simulink model "threePulse"  (Simulink 7.5)
settings: Solver=ode45  StartTime=0.0  StopTime=0.1  RelTol=1e-3
undefined symbols (not defined in the file): deg
libraries: powerlib x14, powerlib_extras x4
settings Model: Creator=Singhal  LastModifiedBy=Singhal

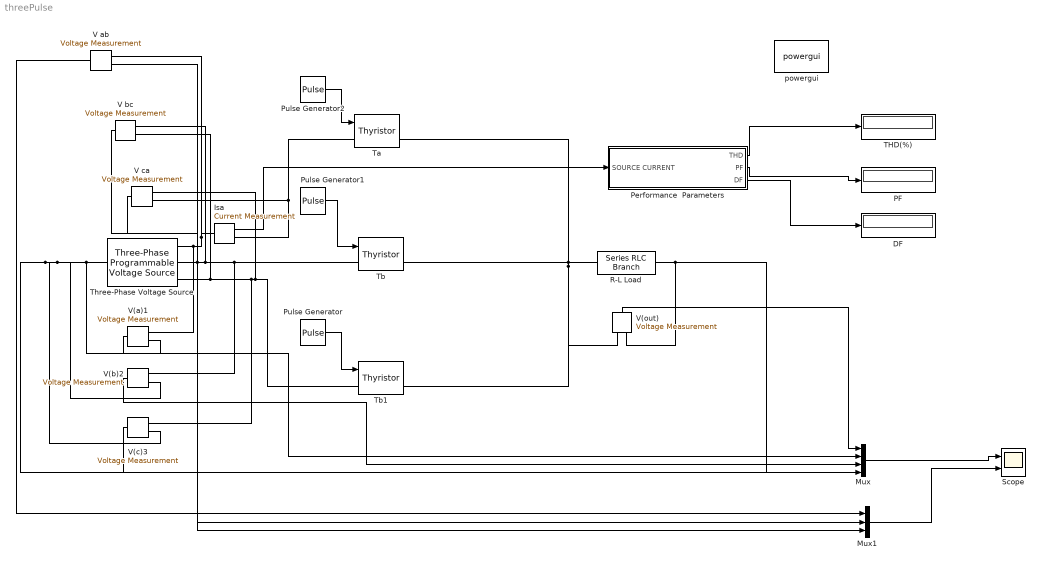
== system threePulse ==
  DF : Display
  Isa : powerlib/Measurements/Current Measurement  DialogController=POWERSYS.PowerSysDialog  SystemSampleTime=-1  PhasorSimulation=off  OutputType=Complex  PSBequivalent=0
  Mux : Mux
  Mux1 : Mux  Inputs=3
  PF : Display
  Performance  Parameters : Subsystem
  Pulse Generator : DiscretePulseGenerator  PulseType=Time based  Amplitude=1  Period=0.02  PulseWidth=5  PhaseDelay=(deg+270)/18000  SampleTime=1
  Pulse Generator1 : DiscretePulseGenerator  PulseType=Time based  Amplitude=1  Period=0.02  PulseWidth=5  PhaseDelay=(deg+150)/18000  SampleTime=1
  Pulse Generator2 : DiscretePulseGenerator  PulseType=Time based  Amplitude=1  Period=0.02  PulseWidth=5  PhaseDelay=(deg+30)/18000  SampleTime=1
  R-L Load : powerlib/Elements/Series RLC Branch  DialogController=POWERSYS.PowerSysDialog  PhysicalDomain=powersysdomain  SubClassName=unknown  LeftPortType=p1  RightPortType=p1  LConnTagsString=__new0  RConnTagsString=__new0  BranchType=RL  Resistance=1  Inductance=1e-3  SetiL0=off  InitialCurrent=0  Capacitance=1e-6  Setx0=off  InitialVoltage=0  Measurements=None
  Scope : Scope  NumInputPorts=2
      settings: YMin=-90~-150  YMax=90~150
  THD(%) : Display
  Ta : powerlib/Power Electronics/Thyristor  DialogController=POWERSYS.PowerSysDialog  SystemSampleTime=-1  Ron=0.001  Lon=0  Vf=0.8  IC=0  Rs=500  Cs=250e-9  Measurements=on
  Tb : powerlib/Power Electronics/Thyristor  DialogController=POWERSYS.PowerSysDialog  SystemSampleTime=-1  Ron=0.001  Lon=0  Vf=0.8  IC=0  Rs=500  Cs=250e-9  Measurements=on
  Tb1 : powerlib/Power Electronics/Thyristor  DialogController=POWERSYS.PowerSysDialog  SystemSampleTime=-1  Ron=0.001  Lon=0  Vf=0.8  IC=0  Rs=500  Cs=250e-9  Measurements=on
  Three-Phase Voltage Source : powerlib/Electrical Sources/Three-Phase Programmable Voltage Source  DialogController=POWERSYS.PowerSysDialog  SystemSampleTime=-1  PositiveSequence="[100  0 50]"  VariationEntity=None  VariationType=Step  VariationStep=0.5  VariationRate=10  VariationMagnitude=0.3  VariationFrequency=2  VariationTiming=[1 2]  VariationPhaseA=off  Amplitudes=[1 0.8 1.2 1.0]  TimeValues=[0 0.1 0.15 0.2]  HarmonicGeneration=off  HarmonicA=[3 0.2 -25 0]  HarmonicB=[2 0.15 35 2]  Timing="[0.05  3]"
  V ab : powerlib/Measurements/Voltage Measurement  DialogController=POWERSYS.PowerSysDialog  SystemSampleTime=-1  PhasorSimulation=off  OutputType=Complex  PSBequivalent=0
  V bc : powerlib/Measurements/Voltage Measurement  DialogController=POWERSYS.PowerSysDialog  SystemSampleTime=-1  PhasorSimulation=off  OutputType=Complex  PSBequivalent=0
  V ca : powerlib/Measurements/Voltage Measurement  DialogController=POWERSYS.PowerSysDialog  SystemSampleTime=-1  PhasorSimulation=off  OutputType=Complex  PSBequivalent=0
  V(a)1 : powerlib/Measurements/Voltage Measurement  DialogController=POWERSYS.PowerSysDialog  SystemSampleTime=-1  PhasorSimulation=off  OutputType=Complex  PSBequivalent=0
  V(b)2 : powerlib/Measurements/Voltage Measurement  DialogController=POWERSYS.PowerSysDialog  SystemSampleTime=-1  PhasorSimulation=off  OutputType=Complex  PSBequivalent=0
  V(c)3 : powerlib/Measurements/Voltage Measurement  DialogController=POWERSYS.PowerSysDialog  SystemSampleTime=-1  PhasorSimulation=off  OutputType=Complex  PSBequivalent=0
  V(out) : powerlib/Measurements/Voltage Measurement  DialogController=POWERSYS.PowerSysDialog  SystemSampleTime=-1  PhasorSimulation=off  OutputType=Complex  PSBequivalent=0
  powergui : powerlib/powergui  Priority=1  SystemSampleTime=-1  SimulationMode=Continuous  SampleTime=50e-6  frequency=60  SPID=off  DisableSnubberDevices=off  DisableRonSwitches=off  DisableVfSwitches=off  SwTol=0  Interpol=off  frequencyindice=50  echomessages=off  HookPort=off  DisplayEquations=off  FunctionMessages=off  EnableUseOfTLC=off  x0status=blocks  RestoreLinks=warning  ResistiveCurrentMeasurement=off  Ylog=off  Xlog=on  ShowGrid=off  save=off  variable=ZData  ZoomFFT=off  StartTime=0.0  cycles=1  DisplayStyle=1  FreqAxis=off  MaxFrequency=1000  frequencyindicesteady=1  display=off  methode=off
  wires:
  Pulse Generator/1 -> Tb1/1
  Pulse Generator1/1 -> Tb/1
  Pulse Generator2/1 -> Ta/1
  Performance  Parameters/2(PF) -> PF/1
  Performance  Parameters/3(DF) -> DF/1
  Performance  Parameters/1(THD) -> THD(%)/1
  Isa/1 -> Performance  Parameters/1(SOURCE CURRENT)
  V(out)/1 -> Mux/1
  V(a)1/1 -> Mux/2
  V(b)2/1 -> Mux/3
  V(c)3/1 -> Mux/4
  Mux/1 -> Scope/1
  V ab/1 -> Mux1/1
  V bc/1 -> Mux1/2
  V ca/1 -> Mux1/3
  Mux1/1 -> Scope/2
  connections:
  Three-Phase Voltage Source/LConn1 -- V(a)1/LConn2 -- V(b)2/LConn2 -- R-L Load/RConn1 -- V(out)/LConn2 -- V(c)3/LConn2
  Tb1/RConn1 -- R-L Load/LConn1 -- Ta/RConn1 -- Tb/RConn1 -- V(out)/LConn1
  Tb/LConn1 -- V(b)2/LConn1 -- Three-Phase Voltage Source/RConn2 -- V ab/LConn2 -- V bc/LConn1
  Tb1/LConn1 -- V(c)3/LConn1 -- Three-Phase Voltage Source/RConn3 -- V bc/LConn2 -- V ca/LConn1
  Isa/LConn1 -- Three-Phase Voltage Source/RConn1 -- V(a)1/LConn1 -- V ab/LConn1
  Isa/RConn1 -- Ta/LConn1 -- V ca/LConn2

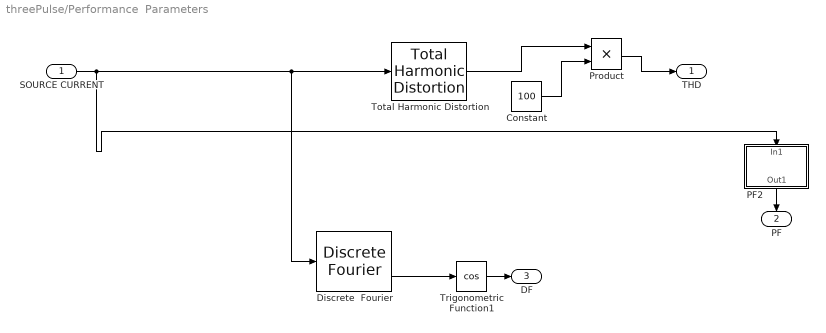
== system threePulse/Performance  Parameters ==
  SOURCE CURRENT : Inport
  Constant : Constant  Value=100  OutDataType=fixdt(1, 16)  OutScaling=2^0
  Discrete  Fourier : powerlib_extras/Discrete Measurements/Discrete  Fourier  DialogController=POWERSYS.PowerSysDialog  SystemSampleTime=-1  Freq=50  n=1  Par_Init=[0 0]  Ts=50e-6
  PF2 : Subsystem
  Product : Product  OutDataType=fixdt(1, 16)  OutScaling=2^0  RndMeth=Zero
  Total Harmonic Distortion : powerlib_extras/Measurements/Total Harmonic Distortion  DialogController=POWERSYS.PowerSysDialog  SystemSampleTime=-1  f1=50
  Trigonometric Function1 : Trigonometry  Operator=cos
  THD : Outport
  PF : Outport  Port=2
  DF : Outport  Port=3
  wires:
  SOURCE CURRENT/1 -> PF2/1(In1), Discrete  Fourier/1, Total Harmonic Distortion/1
  Discrete  Fourier/2 -> Trigonometric Function1/1
  PF2/1(Out1) -> PF/1
  Trigonometric Function1/1 -> DF/1
  Constant/1 -> Product/2
  Total Harmonic Distortion/1 -> Product/1
  Product/1 -> THD/1

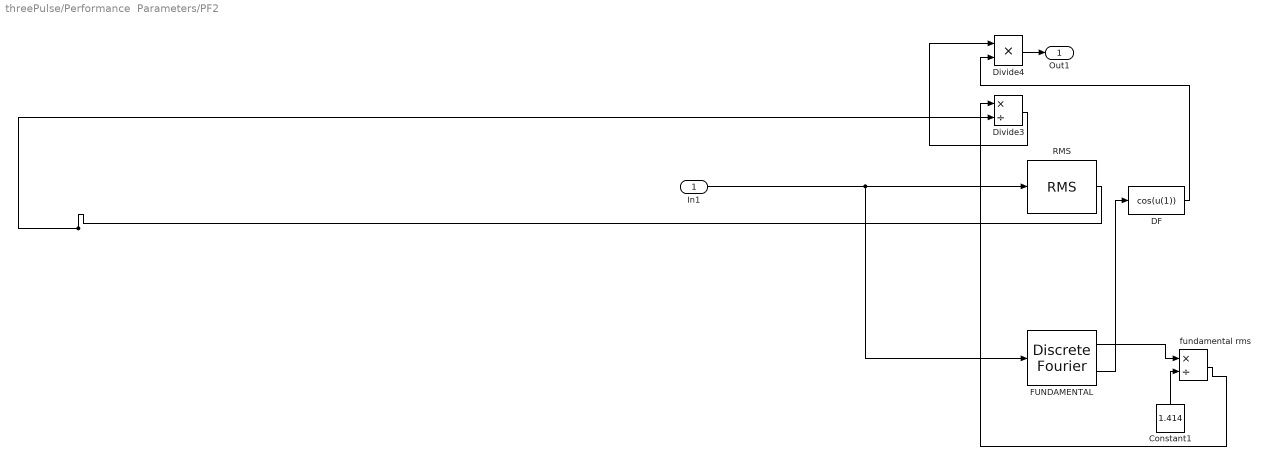
== system threePulse/Performance  Parameters/PF2 ==
  In1 : Inport
  Constant1 : Constant  Value=1.414  OutDataType=fixdt(1, 16)  OutScaling=2^0
  DF : Fcn  Expr=cos(u(1))
  Divide3 : Product  Inputs=*/  OutDataType=fixdt(1, 16)  OutScaling=2^-10
  Divide4 : Product  Inputs=**  OutDataType=fixdt(1, 16)  OutScaling=2^-10
  FUNDAMENTAL : powerlib_extras/Discrete Measurements/Discrete  Fourier  DialogController=POWERSYS.PowerSysDialog  SystemSampleTime=-1  Freq=50  n=1  Par_Init=[0 0]  Ts=50e-3
  RMS : powerlib_extras/Measurements/RMS  DialogController=POWERSYS.PowerSysDialog  SystemSampleTime=-1  f1=50
  fundamental rms : Product  Inputs=*/  OutDataType=fixdt(1, 16)  OutScaling=2^-10
  Out1 : Outport
  wires:
  DF/1 -> Divide4/2
  Divide3/1 -> Divide4/1
  fundamental rms/1 -> Divide3/1
  RMS/1 -> Divide3/2
  FUNDAMENTAL/1 -> fundamental rms/1
  FUNDAMENTAL/2 -> DF/1
  Constant1/1 -> fundamental rms/2
  Divide4/1 -> Out1/1
  In1/1 -> RMS/1, FUNDAMENTAL/1
